simulink model "CruiseControl_pp_harness_ReqProve"  (R2016a)
settings: Solver=ode3  StartTime=0  StopTime=0.40000000000000002  FixedStep=0.10000000000000001  RelTol=1e-3
PreLoadFcn:
  | CruiseControl_dd;
  | definePPenums;
undefined symbols (not defined in the file or in its folder): mintspeed, sigbuilder_block
libraries: sldvlib x20, simulink x8
settings Model: SldvGeneratedHarnessModel=TestUnitModel=CruiseControl_pp|  Creator=The MathWorks Inc.  LastModifiedBy=colosky
settings DataIOCC: LimitDataPoints=on  SaveFormat=StructureWithTime  SaveOutput=off  SaveTime=off
settings OptimizationCC: BlockReduction=off  DefaultParameterBehavior=Inlined  InlineInvariantSignals=on  ExpressionFolding=off  ExpressionDepthLimit=2147483647  InitFltsAndDblsToZero=on  OptimizeModelRefInitCode=on  LifeSpan=1
settings DebuggingCC: SaveWithParameterizedLinksMsg=none  UnderspecifiedInitializationDetection=Classic  MergeDetectMultiDrivingBlocksExec=none  SolverPrmCheckMsg=warning  InheritedTsInSrcMsg=none  FcnCallInpInsideContextMsg=UseLocalSettings  AllowSymbolicDim=off  StateNameClashWarn=warning  StrictBusMsg=ErrorOnBusTreatedAsVector
settings HardwareCC: ProdBitPerPointer=32  ProdLargestAtomicFloat=None  ProdEndianess=Unspecified  ProdWordSize=32  ProdHWDeviceType=32-bit Generic
settings ModelReferenceCC: ModelReferenceNumInstancesAllowed=Single  PropagateSignalLabelsOutOfModel=off
settings SFSimCC: SimParseCustomCode=off
settings RTWCC: SystemTargetFile=ert.tlc  TemplateMakefile=ert_default_tmf  GenerateReport=on  IncludeHyperlinkInReport=on  LaunchReport=on  GenerateTraceInfo=on  GenerateTraceReport=on  GenerateTraceReportSl=on  GenerateTraceReportSf=on  GenerateTraceReportEml=on
settings CodeAppCC: ForceParamTrailComments=on  IgnoreCustomStorageClasses=off  OperatorAnnotations=on  SimulinkDataObjDesc=on  SFDataObjDesc=on  MATLABFcnDesc=on  InsertBlockDesc=on  MATLABSourceComments=on
settings ERTTargetCC: GenerateSampleERTMain=on  InlinedParameterPlacement=NonHierarchical  ERTCustomFileTemplate=example_file_process.tlc
settings ConfigComp: CovMetricSettings=dcme  CovHtmlReporting=off  CovSaveCumulativeToWorkspaceVar=off  CovSaveSingleToWorkspaceVar=off  CovModelRefEnable=Off  CovSFcnEnable=off  DVMode=PropertyProving  DVMaxProcessTime=3000  DVDisplayUnsatisfiableObjectives=on  DVAutomaticStubbing=off  DVMakeOutputFilesUnique=off  DVParameters=on  DVParametersUseConfig=on  DVModelCoverageObjectives=MCDC  DVMaxTestCaseSteps=500  DVTestSuiteOptimization=CombinedObjectives  DVAssertions=EnableAll  DVProofAssumptions=EnableAll  DVDetectIntegerOverflow=off  DVDetectActiveLogic=on  DVMaxViolationSteps=10  DVSaveDataFile=off  DVReportIncludeGraphics=on  DVDisplayResultsOnModel=on

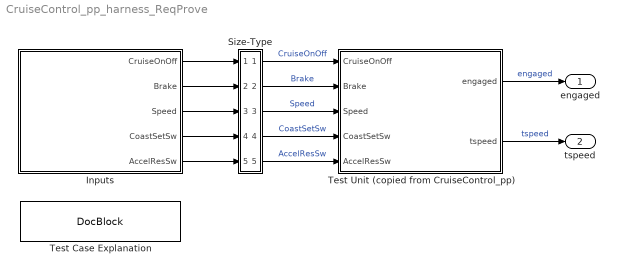
== system CruiseControl_pp_harness_ReqProve ==
  Inputs : Subsystem  Tag=STV Subsys  LoadFcn=sigbuilder_block('load',[50 50 520 400 ]);  StartFcn=sigbuilder_block('start');  StopFcn=sigbuilder_block('stop');  ClipboardFcn=sigbuilder_block('clipboard');  mask(Sigbuilder block){}
      mask init:
      | if ~strcmp(get_param(bdroot(gcb),'SimulationStatus'),'stopped'),tuvar = sigbuilder_block('maskInit'); end
      settings: CopyFcn=sigbuilder_block('copy');  DeleteFcn=sigbuilder_block('delete');  ModelCloseFcn=sigbuilder_block('modelClose');  PreSaveFcn=sigbuilder_block('preSave');  PauseFcn=sigbuilder_block('pause');  ContinueFcn=sigbuilder_block('continue');  NameChangeFcn=sigbuilder_block('namechange');  OpenFcn=sigbuilder_block('open');  CloseFcn=sigbuilder_block('close');
      mask Display: plot(0, 0, 100, 100,[2, 2, 32, 32, 2], [68, 8, 8, 68, 68],[32, 2], [38, 38], [32, 19, 2],[53, 60, 44], [32, 17, 17, 2],[16, 16, 31, 31]);txt = getActiveGroup(gcbh);text(2, 100, txt,'verticalAlignment', 'top');
  Size-Type : Subsystem
  Test Case Explanation : simulink/Model-Wide Utilities/DocBlock  DocumentType=Text
  Test Unit (copied from CruiseControl_pp) : Subsystem
  engaged : Outport  OutDataTypeStr=boolean  PortDimensions=1
  tspeed : Outport  Port=2  OutDataTypeStr=uint8  PortDimensions=1
  wires:
  Inputs/1(CruiseOnOff) -> Size-Type/1(In1)
  Size-Type/1(Out1) -> Test Unit (copied from CruiseControl_pp)/1(CruiseOnOff)  "CruiseOnOff"
  Inputs/2(Brake) -> Size-Type/2(In2)
  Size-Type/2(Out2) -> Test Unit (copied from CruiseControl_pp)/2(Brake)  "Brake"
  Inputs/3(Speed) -> Size-Type/3(In3)
  Size-Type/3(Out3) -> Test Unit (copied from CruiseControl_pp)/3(Speed)  "Speed"
  Inputs/4(CoastSetSw) -> Size-Type/4(In4)
  Size-Type/4(Out4) -> Test Unit (copied from CruiseControl_pp)/4(CoastSetSw)  "CoastSetSw"
  Inputs/5(AccelResSw) -> Size-Type/5(In5)
  Size-Type/5(Out5) -> Test Unit (copied from CruiseControl_pp)/5(AccelResSw)  "AccelResSw"
  Test Unit (copied from CruiseControl_pp)/1(engaged) -> engaged/1  "engaged"
  Test Unit (copied from CruiseControl_pp)/2(tspeed) -> tspeed/1  "tspeed"

== system CruiseControl_pp_harness_ReqProve/Inputs ==
  Demux : Demux  Tag=STV Demux  Outputs=5
  FromWs : FromWorkspace  Tag=STV FromWs  VariableName=tuvar  SampleTime=0
      SigBuilderData=|
      | dataSet.timeRange = [0 0.4]
      | dataSet.name = 'Counterexample 1'
      | sbobj.Name = 'Signal Builder'
      | sbobj.Groups.Name = 'Counterexample 1'
      | sbobj.Groups.Signals(1).Name = 'CruiseOnOff'
      | sbobj.Groups.Signals(1).XData = [0 0.1 0.2 0.3 0.4]
      | sbobj.Groups.Signals(1).YData = [1 1 1 1 1]
      | sbobj.Groups.Signals(2).Name = 'Brake'
      | sbobj.Groups.Signals(2).XData = [0 0.1 0.1 0.2 0.2 0.3 0.3 0.4]
      | sbobj.Groups.Signals(2).YData = [0 0 0 0 0 0 0 0]
      | sbobj.Groups.Signals(3).Name = 'Speed'
      | sbobj.Groups.Signals(3).XData = [0 0.1 0.1 0.2 0.2 0.3 0.3 0.4]
      | sbobj.Groups.Signals(3).YData = [48 48 52 52 27 27 52 52]
      | sbobj.Groups.Signals(4).Name = 'CoastSetSw'
      | sbobj.Groups.Signals(4).XData = [0 0.1 0.1 0.2 0.2 0.3 0.3 0.4]
      | sbobj.Groups.Signals(4).YData = [0 0 0 0 1 1 1 1]
      | sbobj.Groups.Signals(5).Name = 'AccelResSw'
      | sbobj.Groups.Signals(5).XData = [0 0.1 0.1 0.2 0.2 0.3 0.3 0.4]
      | sbobj.Groups.Signals(5).YData = [1 1 1 1 0 0 1 1]
      | sbobj.Groups.TimeRange = [0 0.4]
  CruiseOnOff : Outport  Tag=STV Outport
  Brake : Outport  Tag=STV Outport  Port=2
  Speed : Outport  Tag=STV Outport  Port=3
  CoastSetSw : Outport  Tag=STV Outport  Port=4
  AccelResSw : Outport  Tag=STV Outport  Port=5
  wires:
  FromWs/1 -> Demux/1
  Demux/1 -> CruiseOnOff/1
  Demux/2 -> Brake/1
  Demux/3 -> Speed/1
  Demux/4 -> CoastSetSw/1
  Demux/5 -> AccelResSw/1

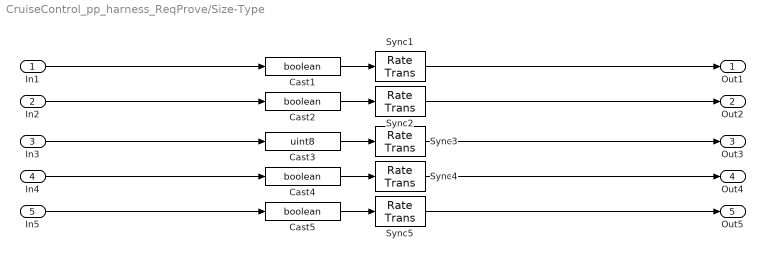
== system CruiseControl_pp_harness_ReqProve/Size-Type ==
  In1 : Inport
  In2 : Inport  Port=2
  In3 : Inport  Port=3
  In4 : Inport  Port=4
  In5 : Inport  Port=5
  Cast{1..2,4..5} (4 alike) : DataTypeConversion  OutDataTypeStr=boolean  RndMeth=Nearest  SaturateOnIntegerOverflow=on
  Cast3 : DataTypeConversion  OutDataTypeStr=uint8  RndMeth=Nearest  SaturateOnIntegerOverflow=on
  Sync{1..5} (5 alike) : RateTransition  OutPortSampleTime=[0.10000000000000001,0]
  Out1 : Outport
  Out2 : Outport  Port=2
  Out3 : Outport  Port=3
  Out4 : Outport  Port=4
  Out5 : Outport  Port=5
  wires:
  In1/1 -> Cast1/1
  Cast1/1 -> Sync1/1
  Sync1/1 -> Out1/1
  In2/1 -> Cast2/1
  Cast2/1 -> Sync2/1
  Sync2/1 -> Out2/1
  In3/1 -> Cast3/1
  Cast3/1 -> Sync3/1
  Sync3/1 -> Out3/1
  In4/1 -> Cast4/1
  Cast4/1 -> Sync4/1
  Sync4/1 -> Out4/1
  In5/1 -> Cast5/1
  Cast5/1 -> Sync5/1
  Sync5/1 -> Out5/1

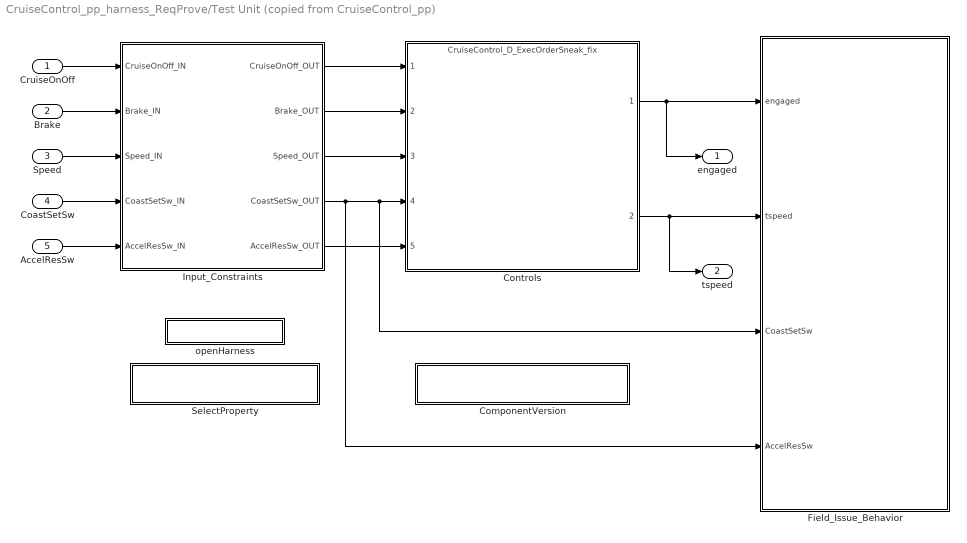
== system CruiseControl_pp_harness_ReqProve/Test Unit (copied from CruiseControl_pp) ==
  CruiseOnOff : Inport  OutDataTypeStr=boolean  PortDimensions=1
  Brake : Inport  Port=2  OutDataTypeStr=boolean  PortDimensions=1
  Speed : Inport  Port=3  OutDataTypeStr=uint8  PortDimensions=1
  CoastSetSw : Inport  Port=4  OutDataTypeStr=boolean  PortDimensions=1
  AccelResSw : Inport  Port=5  OutDataTypeStr=boolean  PortDimensions=1
  ComponentVersion : Subsystem  mask(ControlsVersion){}
      mask help: Selects the block choice for the "Controls" subystem.
      settings: OpenFcn=|
      | [~,enumVers] = enumeration('CtrlsVerEnum');
      | [selection, ok] = listdlg('Name','Component Version','ListSize',[210 110],'SelectionMode','single', ...
      |    'PromptString','Select Cruise Control version...','ListString',enumVers,'InitialValue',uint32(CtrlsVer));
      | waitfor(selection);
      | if ok
      |    CtrlsVer = CtrlsVerEnum(enumVers{selection});
      | end
      mask Display: disp('Select Cruise Control version to verify...');
  Controls : ModelReference  ModelNameDialog=CruiseControl_D_ExecOrderSneak_fix.slx  SimulationMode=Normal  Variant=on  ModelReferenceVersion=1.515
  Field_Issue_Behavior : Subsystem  Variant=on
      settings: AttributesFormatString=%<BlockChoice>
  Input_Constraints : Subsystem  Variant=on
      settings: AttributesFormatString=%<BlockChoice>
  SelectProperty : Subsystem  mask(PropertySelection){}
      mask help: Selects the block choice for the "Input_Constraints" and "Field_Issue_Behavior" subystems.
      settings: OpenFcn=|
      | [~,enumProps] = enumeration('PropEnum');
      | [selection, ok] = listdlg('Name','Propery To Prove','ListSize',[210 110],'SelectionMode','single', ...
      |    'PromptString','Select Property to Prove...','ListString',enumProps,'InitialValue',uint32(Prop2Prove));
      | waitfor(selection);
      | if ok
      |    Prop2Prove = PropEnum(enumProps{selection});
      | end
      mask DialogControl DescGroupVar Prompt: Description
      mask Display: disp('Selected Property to Prove...');
  openHarness : Subsystem
      settings: OpenFcn=|
      | switch (CtrlsVer)
      | case CtrlsVerEnum.CtrlC_ExecOrder_fix
      |     load_PP_harness('CruiseControl_pp_harness_FieldIssue');
      | case CtrlsVerEnum.CtrlD_ExecOrderSneak_fix
      |     load_PP_harness('CruiseControl_pp_harness_ReqProve');
      | case CtrlsVerEnum.CtrlE_ExecOrderSneakDblReject_fix
      |     load_PP_harness('CruiseControl_pp_harness_ReqWithParsProve');
      | end
      mask Display: disp(['Open Harness']);
  engaged : Outport  OutDataTypeStr=boolean  PortDimensions=1
  tspeed : Outport  Port=2  OutDataTypeStr=uint8  PortDimensions=1
  wires:
  Controls/2 -> Field_Issue_Behavior/2(tspeed), tspeed/1
  AccelResSw/1 -> Input_Constraints/5(AccelResSw_IN)
  Speed/1 -> Input_Constraints/3(Speed_IN)
  CruiseOnOff/1 -> Input_Constraints/1(CruiseOnOff_IN)
  Brake/1 -> Input_Constraints/2(Brake_IN)
  CoastSetSw/1 -> Input_Constraints/4(CoastSetSw_IN)
  Input_Constraints/1(CruiseOnOff_OUT) -> Controls/1
  Input_Constraints/2(Brake_OUT) -> Controls/2
  Input_Constraints/3(Speed_OUT) -> Controls/3
  Input_Constraints/4(CoastSetSw_OUT) -> Controls/4, Field_Issue_Behavior/3(CoastSetSw), Field_Issue_Behavior/4(AccelResSw)
  Input_Constraints/5(AccelResSw_OUT) -> Controls/5
  Controls/1 -> Field_Issue_Behavior/1(engaged), engaged/1

== system CruiseControl_pp_harness_ReqProve/Test Unit (copied from CruiseControl_pp)/ComponentVersion ==

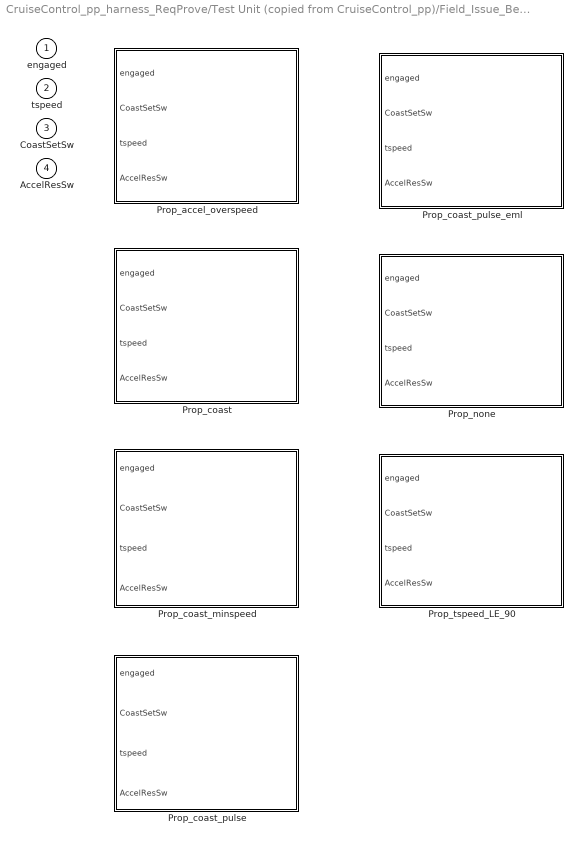
== system CruiseControl_pp_harness_ReqProve/Test Unit (copied from CruiseControl_pp)/Field_Issue_Behavior ==
  engaged : Inport
  tspeed : Inport  Port=2
  CoastSetSw : Inport  Port=3
  AccelResSw : Inport  Port=4
  Prop_accel_overspeed : Subsystem  VariantControl=Prop2Prove == PropEnum.Prop_accel_overspeed
  Prop_coast : Subsystem  VariantControl=Prop2Prove == PropEnum.Prop_coast
  Prop_coast_minspeed : Subsystem  VariantControl=Prop2Prove == PropEnum.Prop_coast_minspeed
  Prop_coast_pulse : Subsystem  VariantControl=Prop2Prove == PropEnum.Prop_coast_pulse
  Prop_coast_pulse_eml : Subsystem  VariantControl=Prop2Prove == PropEnum.Prop_coast_pulse_eml
  Prop_none : Subsystem  VariantControl=Prop2Prove == PropEnum.Prop_none
  Prop_tspeed_LE_90 : Subsystem  VariantControl=Prop2Prove == PropEnum.Prop_tspeed_LE_90

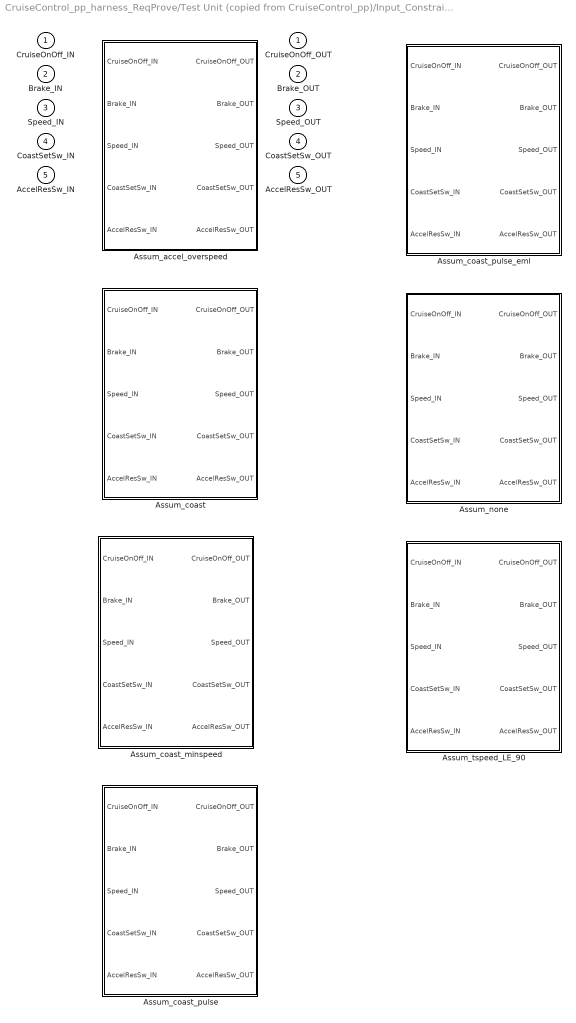
== system CruiseControl_pp_harness_ReqProve/Test Unit (copied from CruiseControl_pp)/Input_Constraints ==
  CruiseOnOff_IN : Inport
  Brake_IN : Inport  Port=2
  Speed_IN : Inport  Port=3
  CoastSetSw_IN : Inport  Port=4
  AccelResSw_IN : Inport  Port=5
  Assum_accel_overspeed : Subsystem  VariantControl=Prop2Prove == PropEnum.Prop_accel_overspeed
  Assum_coast : Subsystem  VariantControl=Prop2Prove == PropEnum.Prop_coast
  Assum_coast_minspeed : Subsystem  VariantControl=Prop2Prove == PropEnum.Prop_coast_minspeed
  Assum_coast_pulse : Subsystem  VariantControl=Prop2Prove == PropEnum.Prop_coast_pulse
  Assum_coast_pulse_eml : Subsystem  VariantControl=Prop2Prove == PropEnum.Prop_coast_pulse_eml
  Assum_none : Subsystem  VariantControl=Prop2Prove == PropEnum.Prop_none
  Assum_tspeed_LE_90 : Subsystem  VariantControl=Prop2Prove == PropEnum.Prop_tspeed_LE_90
  CruiseOnOff_OUT : Outport
  Brake_OUT : Outport  Port=2
  Speed_OUT : Outport  Port=3
  CoastSetSw_OUT : Outport  Port=4
  AccelResSw_OUT : Outport  Port=5

== system CruiseControl_pp_harness_ReqProve/Test Unit (copied from CruiseControl_pp)/SelectProperty ==

== system CruiseControl_pp_harness_ReqProve/Test Unit (copied from CruiseControl_pp)/openHarness ==

== system CruiseControl_pp_harness_ReqProve/Test Unit (copied from CruiseControl_pp)/Field_Issue_Behavior/Prop_accel_overspeed ==
  engaged : Inport
  CoastSetSw : Inport  Port=2
  tspeed : Inport  Port=3
  AccelResSw : Inport  Port=4
  Compare To Constant : simulink/Logic and Bit Operations/Compare To Constant  relop=<=  const=95  OutDataTypeStr=boolean
  EngagedImplies : sldvlib/Verification Utilities/Implies
  Logical Operator2 : Logic  AllPortsSameDT=off  OutDataTypeStr=boolean
  Prop_accel_overspeed : sldvlib/Objectives and Constraints/Proof Objective  enabled=on  customAVTBlockType=Proof Objective  intervals=true  dispValues=on  outEnabled=off  enableStopSim=off
      settings: AttributesFormatString=%<intervals>
  Terminator1 : Terminator
  wires:
  EngagedImplies/1 -> Prop_accel_overspeed/1
  Logical Operator2/1 -> EngagedImplies/1
  AccelResSw/1 -> Logical Operator2/2
  engaged/1 -> Logical Operator2/1
  Compare To Constant/1 -> EngagedImplies/2
  tspeed/1 -> Compare To Constant/1
  CoastSetSw/1 -> Terminator1/1

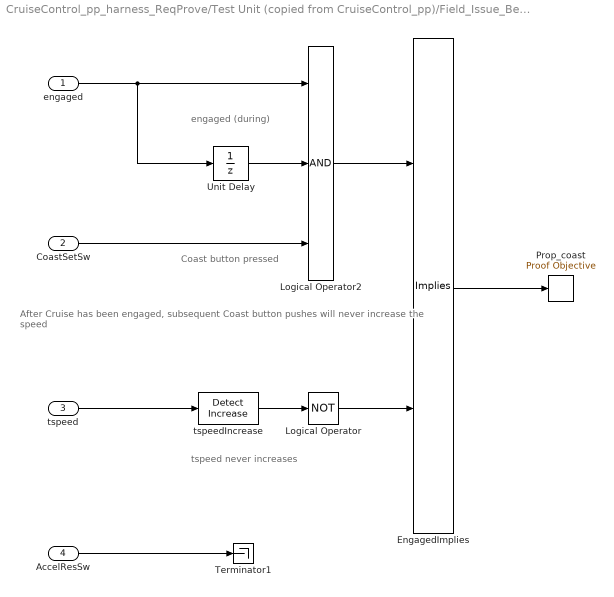
== system CruiseControl_pp_harness_ReqProve/Test Unit (copied from CruiseControl_pp)/Field_Issue_Behavior/Prop_coast ==
  note: After Cruise has been engaged, subsequent Coast button pushes will never increase the speed
  note: Coast button pressed
  note: tspeed never increases
  note: engaged (during)
  engaged : Inport
  CoastSetSw : Inport  Port=2
  tspeed : Inport  Port=3
  AccelResSw : Inport  Port=4
  EngagedImplies : sldvlib/Verification Utilities/Implies
  Logical Operator : Logic  Operator=NOT  AllPortsSameDT=off  OutDataTypeStr=boolean
  Logical Operator2 : Logic  Inputs=3  AllPortsSameDT=off  OutDataTypeStr=boolean
  Prop_coast : sldvlib/Objectives and Constraints/Proof Objective  enabled=on  customAVTBlockType=Proof Objective  intervals=true  dispValues=on  outEnabled=off  enableStopSim=off
      settings: AttributesFormatString=%<intervals>
  Terminator1 : Terminator
  Unit Delay : UnitDelay  SampleTime=-1
  tspeedIncrease : simulink/Logic and Bit Operations/Detect Increase  vinit=0.0  InputProcessing=Inherited  OutDataTypeStr=boolean
  wires:
  EngagedImplies/1 -> Prop_coast/1
  tspeedIncrease/1 -> Logical Operator/1
  tspeed/1 -> tspeedIncrease/1
  Unit Delay/1 -> Logical Operator2/2
  AccelResSw/1 -> Terminator1/1
  engaged/1 -> Logical Operator2/1, Unit Delay/1
  Logical Operator/1 -> EngagedImplies/2
  CoastSetSw/1 -> Logical Operator2/3
  Logical Operator2/1 -> EngagedImplies/1

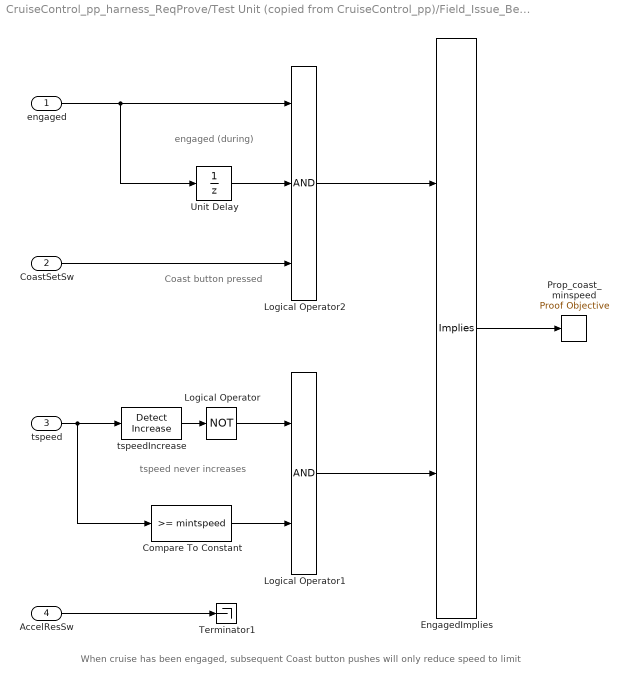
== system CruiseControl_pp_harness_ReqProve/Test Unit (copied from CruiseControl_pp)/Field_Issue_Behavior/Prop_coast_minspeed ==
  note: When cruise has been engaged, subsequent Coast button pushes will only reduce speed to limit
  note: Coast button pressed
  note: tspeed never increases
  note: engaged (during)
  engaged : Inport
  CoastSetSw : Inport  Port=2
  tspeed : Inport  Port=3
  AccelResSw : Inport  Port=4
  Compare To Constant : simulink/Logic and Bit Operations/Compare To Constant  relop=>=  const=mintspeed  OutDataTypeStr=boolean
  EngagedImplies : sldvlib/Verification Utilities/Implies
  Logical Operator : Logic  Operator=NOT  AllPortsSameDT=off  OutDataTypeStr=boolean
  Logical Operator1 : Logic  AllPortsSameDT=off  OutDataTypeStr=boolean
  Logical Operator2 : Logic  Inputs=3  AllPortsSameDT=off  OutDataTypeStr=boolean
  Prop_coast_minspeed : sldvlib/Objectives and Constraints/Proof Objective  enabled=on  customAVTBlockType=Proof Objective  intervals=true  dispValues=on  outEnabled=off  enableStopSim=off
      settings: AttributesFormatString=%<intervals>
  Terminator1 : Terminator
  Unit Delay : UnitDelay  SampleTime=-1
  tspeedIncrease : simulink/Logic and Bit Operations/Detect Increase  vinit=0.0  InputProcessing=Inherited  OutDataTypeStr=boolean
  wires:
  Logical Operator1/1 -> EngagedImplies/2
  Compare To Constant/1 -> Logical Operator1/2
  Logical Operator/1 -> Logical Operator1/1
  EngagedImplies/1 -> Prop_coast_minspeed/1
  tspeedIncrease/1 -> Logical Operator/1
  tspeed/1 -> tspeedIncrease/1, Compare To Constant/1
  Unit Delay/1 -> Logical Operator2/2
  AccelResSw/1 -> Terminator1/1
  engaged/1 -> Logical Operator2/1, Unit Delay/1
  CoastSetSw/1 -> Logical Operator2/3
  Logical Operator2/1 -> EngagedImplies/1

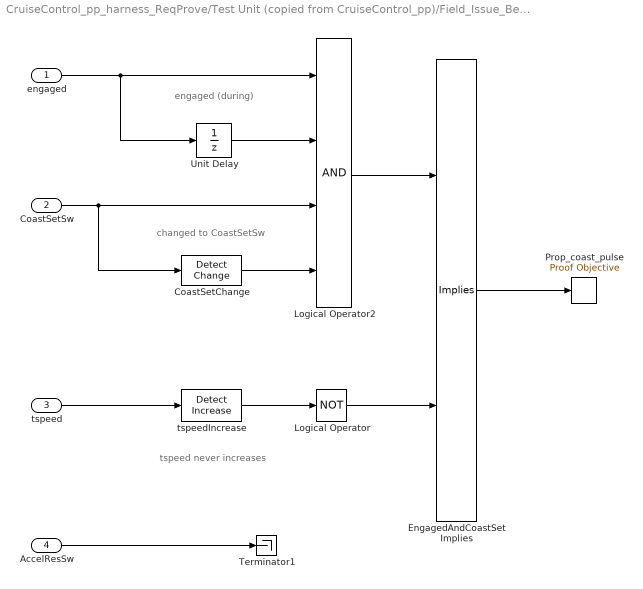
== system CruiseControl_pp_harness_ReqProve/Test Unit (copied from CruiseControl_pp)/Field_Issue_Behavior/Prop_coast_pulse ==
  note: engaged (during)
  note: tspeed never increases
  note: changed to CoastSetSw
  engaged : Inport
  CoastSetSw : Inport  Port=2
  tspeed : Inport  Port=3
  AccelResSw : Inport  Port=4
  CoastSetChange : simulink/Logic and Bit Operations/Detect Change  vinit=0  InputProcessing=Inherited  OutDataTypeStr=boolean
  EngagedAndCoastSetImplies : sldvlib/Verification Utilities/Implies
  Logical Operator : Logic  Operator=NOT  AllPortsSameDT=off  OutDataTypeStr=boolean
  Logical Operator2 : Logic  Inputs=4  AllPortsSameDT=off  OutDataTypeStr=boolean
  Prop_coast_pulse : sldvlib/Objectives and Constraints/Proof Objective  enabled=on  customAVTBlockType=Proof Objective  intervals=true  dispValues=on  outEnabled=off  enableStopSim=off
      settings: AttributesFormatString=%<intervals>
  Terminator1 : Terminator
  Unit Delay : UnitDelay  SampleTime=-1
  tspeedIncrease : simulink/Logic and Bit Operations/Detect Increase  vinit=0.0  InputProcessing=Inherited  OutDataTypeStr=boolean
  wires:
  CoastSetChange/1 -> Logical Operator2/4
  Unit Delay/1 -> Logical Operator2/2
  engaged/1 -> Logical Operator2/1, Unit Delay/1
  EngagedAndCoastSetImplies/1 -> Prop_coast_pulse/1
  tspeedIncrease/1 -> Logical Operator/1
  AccelResSw/1 -> Terminator1/1
  Logical Operator2/1 -> EngagedAndCoastSetImplies/1
  tspeed/1 -> tspeedIncrease/1
  CoastSetSw/1 -> CoastSetChange/1, Logical Operator2/3
  Logical Operator/1 -> EngagedAndCoastSetImplies/2

== system CruiseControl_pp_harness_ReqProve/Test Unit (copied from CruiseControl_pp)/Field_Issue_Behavior/Prop_coast_pulse_eml ==
  engaged : Inport
  CoastSetSw : Inport  Port=2
  tspeed : Inport  Port=3
  AccelResSw : Inport  Port=4
  MATLAB Function : Subsystem  TreatAsAtomicUnit=on
  Porp_coast_pulse_eml : sldvlib/Objectives and Constraints/Proof Objective  enabled=on  customAVTBlockType=Proof Objective  intervals=true  dispValues=on  outEnabled=off  enableStopSim=off
      settings: AttributesFormatString=%<intervals>
  Terminator1 : Terminator
  wires:
  MATLAB Function/1(property) -> Porp_coast_pulse_eml/1
  tspeed/1 -> MATLAB Function/3(tspeed)
  CoastSetSw/1 -> MATLAB Function/2(CoastSetSw)
  engaged/1 -> MATLAB Function/1(engaged)
  AccelResSw/1 -> Terminator1/1

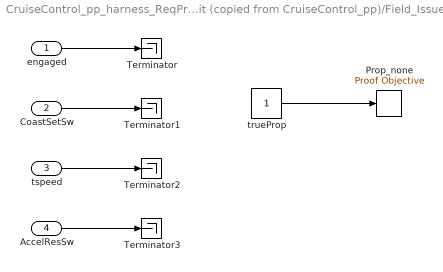
== system CruiseControl_pp_harness_ReqProve/Test Unit (copied from CruiseControl_pp)/Field_Issue_Behavior/Prop_none ==
  engaged : Inport
  CoastSetSw : Inport  Port=2
  tspeed : Inport  Port=3
  AccelResSw : Inport  Port=4
  Prop_none : sldvlib/Objectives and Constraints/Proof Objective  enabled=on  customAVTBlockType=Proof Objective  intervals=true  dispValues=on  outEnabled=off  enableStopSim=off
      settings: AttributesFormatString=%<intervals>
  Terminator{,1..3} (4 alike) : Terminator
  trueProp : Constant  OutDataTypeStr=boolean
  wires:
  trueProp/1 -> Prop_none/1
  AccelResSw/1 -> Terminator3/1
  engaged/1 -> Terminator/1
  tspeed/1 -> Terminator2/1
  CoastSetSw/1 -> Terminator1/1

== system CruiseControl_pp_harness_ReqProve/Test Unit (copied from CruiseControl_pp)/Field_Issue_Behavior/Prop_tspeed_LE_90 ==
  engaged : Inport
  CoastSetSw : Inport  Port=2
  tspeed : Inport  Port=3
  AccelResSw : Inport  Port=4
  Compare To Constant : simulink/Logic and Bit Operations/Compare To Constant  relop=<=  const=90  OutDataTypeStr=boolean
  Prop_tspeed_LE_90 : sldvlib/Objectives and Constraints/Proof Objective  enabled=on  customAVTBlockType=Proof Objective  intervals=true  dispValues=on  outEnabled=off  enableStopSim=off
      settings: AttributesFormatString=%<intervals>
  Terminator : Terminator
  Terminator1 : Terminator
  Terminator2 : Terminator
  wires:
  Compare To Constant/1 -> Prop_tspeed_LE_90/1
  AccelResSw/1 -> Terminator2/1
  CoastSetSw/1 -> Terminator1/1
  tspeed/1 -> Compare To Constant/1
  engaged/1 -> Terminator/1

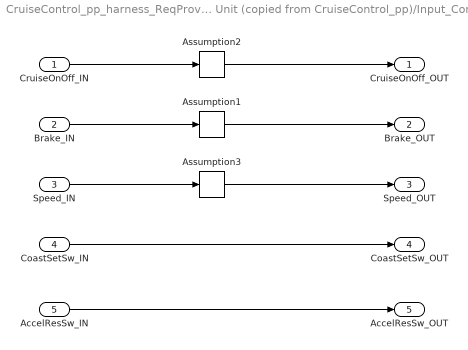
== system CruiseControl_pp_harness_ReqProve/Test Unit (copied from CruiseControl_pp)/Input_Constraints/Assum_accel_overspeed ==
  CruiseOnOff_IN : Inport  OutDataTypeStr=boolean  PortDimensions=1
  Brake_IN : Inport  Port=2  OutDataTypeStr=boolean  PortDimensions=1
  Speed_IN : Inport  Port=3  OutDataTypeStr=uint8  PortDimensions=1
  CoastSetSw_IN : Inport  Port=4  OutDataTypeStr=boolean  PortDimensions=1
  AccelResSw_IN : Inport  Port=5  OutDataTypeStr=boolean  PortDimensions=1
  Assumption1 : sldvlib/Objectives and Constraints/Assumption  enabled=on  customAVTBlockType=Assumption  intervals=false  initial=off  dispValues=on  outEnabled=on
      settings: AttributesFormatString=%<intervals>
  Assumption2 : sldvlib/Objectives and Constraints/Assumption  enabled=on  customAVTBlockType=Assumption  intervals=true  initial=off  dispValues=on  outEnabled=on
      settings: AttributesFormatString=%<intervals>
  Assumption3 : sldvlib/Objectives and Constraints/Assumption  enabled=on  customAVTBlockType=Assumption  intervals={[88 Inf]}  initial=off  dispValues=on  outEnabled=on
      settings: AttributesFormatString=%<intervals>
  CruiseOnOff_OUT : Outport
  Brake_OUT : Outport  Port=2
  Speed_OUT : Outport  Port=3
  CoastSetSw_OUT : Outport  Port=4
  AccelResSw_OUT : Outport  Port=5
  wires:
  Assumption3/1 -> Speed_OUT/1
  Assumption1/1 -> Brake_OUT/1
  Assumption2/1 -> CruiseOnOff_OUT/1
  CruiseOnOff_IN/1 -> Assumption2/1
  Brake_IN/1 -> Assumption1/1
  AccelResSw_IN/1 -> AccelResSw_OUT/1
  CoastSetSw_IN/1 -> CoastSetSw_OUT/1
  Speed_IN/1 -> Assumption3/1

== system CruiseControl_pp_harness_ReqProve/Test Unit (copied from CruiseControl_pp)/Input_Constraints/Assum_coast ==
  CruiseOnOff_IN : Inport  OutDataTypeStr=boolean  PortDimensions=1
  Brake_IN : Inport  Port=2  OutDataTypeStr=boolean  PortDimensions=1
  Speed_IN : Inport  Port=3  OutDataTypeStr=uint8  PortDimensions=1
  CoastSetSw_IN : Inport  Port=4  OutDataTypeStr=boolean  PortDimensions=1
  AccelResSw_IN : Inport  Port=5  OutDataTypeStr=boolean  PortDimensions=1
  CruiseOnOff_OUT : Outport
  Brake_OUT : Outport  Port=2
  Speed_OUT : Outport  Port=3
  CoastSetSw_OUT : Outport  Port=4
  AccelResSw_OUT : Outport  Port=5
  wires:
  AccelResSw_IN/1 -> AccelResSw_OUT/1
  Brake_IN/1 -> Brake_OUT/1
  CruiseOnOff_IN/1 -> CruiseOnOff_OUT/1
  Speed_IN/1 -> Speed_OUT/1
  CoastSetSw_IN/1 -> CoastSetSw_OUT/1

== system CruiseControl_pp_harness_ReqProve/Test Unit (copied from CruiseControl_pp)/Input_Constraints/Assum_coast_minspeed ==
  CruiseOnOff_IN : Inport  OutDataTypeStr=boolean  PortDimensions=1
  Brake_IN : Inport  Port=2  OutDataTypeStr=boolean  PortDimensions=1
  Speed_IN : Inport  Port=3  OutDataTypeStr=uint8  PortDimensions=1
  CoastSetSw_IN : Inport  Port=4  OutDataTypeStr=boolean  PortDimensions=1
  AccelResSw_IN : Inport  Port=5  OutDataTypeStr=boolean  PortDimensions=1
  CruiseOnOff_OUT : Outport
  Brake_OUT : Outport  Port=2
  Speed_OUT : Outport  Port=3
  CoastSetSw_OUT : Outport  Port=4
  AccelResSw_OUT : Outport  Port=5
  wires:
  AccelResSw_IN/1 -> AccelResSw_OUT/1
  Brake_IN/1 -> Brake_OUT/1
  CruiseOnOff_IN/1 -> CruiseOnOff_OUT/1
  Speed_IN/1 -> Speed_OUT/1
  CoastSetSw_IN/1 -> CoastSetSw_OUT/1

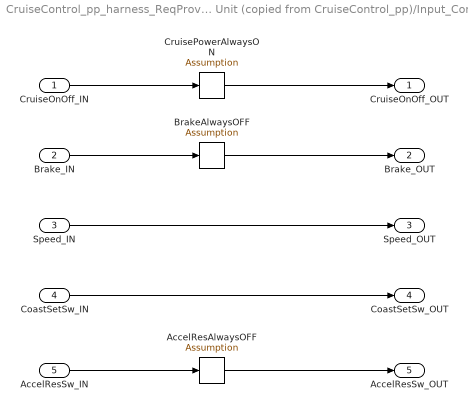
== system CruiseControl_pp_harness_ReqProve/Test Unit (copied from CruiseControl_pp)/Input_Constraints/Assum_coast_pulse ==
  CruiseOnOff_IN : Inport  OutDataTypeStr=boolean  PortDimensions=1
  Brake_IN : Inport  Port=2  OutDataTypeStr=boolean  PortDimensions=1
  Speed_IN : Inport  Port=3  OutDataTypeStr=uint8  PortDimensions=1
  CoastSetSw_IN : Inport  Port=4  OutDataTypeStr=boolean  PortDimensions=1
  AccelResSw_IN : Inport  Port=5  OutDataTypeStr=boolean  PortDimensions=1
  AccelResAlwaysOFF : sldvlib/Objectives and Constraints/Assumption  enabled=on  customAVTBlockType=Assumption  intervals=false  initial=off  dispValues=on  outEnabled=on
      settings: AttributesFormatString=%<intervals>
  BrakeAlwaysOFF : sldvlib/Objectives and Constraints/Assumption  enabled=on  customAVTBlockType=Assumption  intervals=false  initial=off  dispValues=on  outEnabled=on
      settings: AttributesFormatString=%<intervals>
  CruisePowerAlwaysON : sldvlib/Objectives and Constraints/Assumption  enabled=on  customAVTBlockType=Assumption  intervals=true  initial=off  dispValues=on  outEnabled=on
      settings: AttributesFormatString=%<intervals>
  CruiseOnOff_OUT : Outport
  Brake_OUT : Outport  Port=2
  Speed_OUT : Outport  Port=3
  CoastSetSw_OUT : Outport  Port=4
  AccelResSw_OUT : Outport  Port=5
  wires:
  CoastSetSw_IN/1 -> CoastSetSw_OUT/1
  AccelResSw_IN/1 -> AccelResAlwaysOFF/1
  Speed_IN/1 -> Speed_OUT/1
  Brake_IN/1 -> BrakeAlwaysOFF/1
  CruiseOnOff_IN/1 -> CruisePowerAlwaysON/1
  CruisePowerAlwaysON/1 -> CruiseOnOff_OUT/1
  BrakeAlwaysOFF/1 -> Brake_OUT/1
  AccelResAlwaysOFF/1 -> AccelResSw_OUT/1

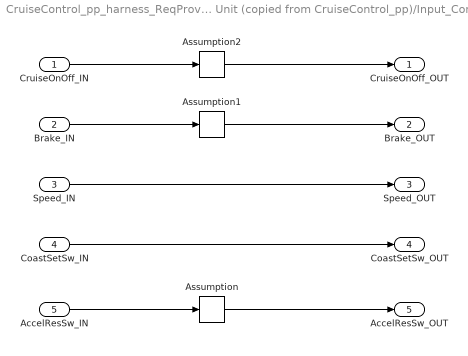
== system CruiseControl_pp_harness_ReqProve/Test Unit (copied from CruiseControl_pp)/Input_Constraints/Assum_coast_pulse_eml ==
  CruiseOnOff_IN : Inport  OutDataTypeStr=boolean  PortDimensions=1
  Brake_IN : Inport  Port=2  OutDataTypeStr=boolean  PortDimensions=1
  Speed_IN : Inport  Port=3  OutDataTypeStr=uint8  PortDimensions=1
  CoastSetSw_IN : Inport  Port=4  OutDataTypeStr=boolean  PortDimensions=1
  AccelResSw_IN : Inport  Port=5  OutDataTypeStr=boolean  PortDimensions=1
  Assumption : sldvlib/Objectives and Constraints/Assumption  enabled=on  customAVTBlockType=Assumption  intervals=false  initial=off  dispValues=on  outEnabled=on
      settings: AttributesFormatString=%<intervals>
  Assumption1 : sldvlib/Objectives and Constraints/Assumption  enabled=on  customAVTBlockType=Assumption  intervals=false  initial=off  dispValues=on  outEnabled=on
      settings: AttributesFormatString=%<intervals>
  Assumption2 : sldvlib/Objectives and Constraints/Assumption  enabled=on  customAVTBlockType=Assumption  intervals=true  initial=off  dispValues=on  outEnabled=on
      settings: AttributesFormatString=%<intervals>
  CruiseOnOff_OUT : Outport
  Brake_OUT : Outport  Port=2
  Speed_OUT : Outport  Port=3
  CoastSetSw_OUT : Outport  Port=4
  AccelResSw_OUT : Outport  Port=5
  wires:
  Assumption/1 -> AccelResSw_OUT/1
  Assumption1/1 -> Brake_OUT/1
  Assumption2/1 -> CruiseOnOff_OUT/1
  CruiseOnOff_IN/1 -> Assumption2/1
  Brake_IN/1 -> Assumption1/1
  Speed_IN/1 -> Speed_OUT/1
  AccelResSw_IN/1 -> Assumption/1
  CoastSetSw_IN/1 -> CoastSetSw_OUT/1

== system CruiseControl_pp_harness_ReqProve/Test Unit (copied from CruiseControl_pp)/Input_Constraints/Assum_none ==
  CruiseOnOff_IN : Inport  OutDataTypeStr=boolean  PortDimensions=1
  Brake_IN : Inport  Port=2  OutDataTypeStr=boolean  PortDimensions=1
  Speed_IN : Inport  Port=3  OutDataTypeStr=uint8  PortDimensions=1
  CoastSetSw_IN : Inport  Port=4  OutDataTypeStr=boolean  PortDimensions=1
  AccelResSw_IN : Inport  Port=5  OutDataTypeStr=boolean  PortDimensions=1
  CruiseOnOff_OUT : Outport
  Brake_OUT : Outport  Port=2
  Speed_OUT : Outport  Port=3
  CoastSetSw_OUT : Outport  Port=4
  AccelResSw_OUT : Outport  Port=5
  wires:
  CruiseOnOff_IN/1 -> CruiseOnOff_OUT/1
  Brake_IN/1 -> Brake_OUT/1
  Speed_IN/1 -> Speed_OUT/1
  AccelResSw_IN/1 -> AccelResSw_OUT/1
  CoastSetSw_IN/1 -> CoastSetSw_OUT/1

== system CruiseControl_pp_harness_ReqProve/Test Unit (copied from CruiseControl_pp)/Input_Constraints/Assum_tspeed_LE_90 ==
  CruiseOnOff_IN : Inport  OutDataTypeStr=boolean  PortDimensions=1
  Brake_IN : Inport  Port=2  OutDataTypeStr=boolean  PortDimensions=1
  Speed_IN : Inport  Port=3  OutDataTypeStr=uint8  PortDimensions=1
  CoastSetSw_IN : Inport  Port=4  OutDataTypeStr=boolean  PortDimensions=1
  AccelResSw_IN : Inport  Port=5  OutDataTypeStr=boolean  PortDimensions=1
  CruiseOnOff_OUT : Outport
  Brake_OUT : Outport  Port=2
  Speed_OUT : Outport  Port=3
  CoastSetSw_OUT : Outport  Port=4
  AccelResSw_OUT : Outport  Port=5
  wires:
  Speed_IN/1 -> Speed_OUT/1
  CoastSetSw_IN/1 -> CoastSetSw_OUT/1
  AccelResSw_IN/1 -> AccelResSw_OUT/1
  Brake_IN/1 -> Brake_OUT/1
  CruiseOnOff_IN/1 -> CruiseOnOff_OUT/1

== system CruiseControl_pp_harness_ReqProve/Test Unit (copied from CruiseControl_pp)/Field_Issue_Behavior/Prop_coast_pulse_eml/MATLAB Function ==
  engaged : Inport
  CoastSetSw : Inport  Port=2
  tspeed : Inport  Port=3
  " Demux " : Demux  Outputs=1
  " SFunction " : S-Function  Tag=Stateflow S-Function propertyLib 2  FunctionName=sf_sfun  PortCounts=[3 2]  SFunctionDeploymentMode=off  EnableBusSupport=off
  " Terminator " : Terminator
  property : Outport
  wires:
  " SFunction "/1 -> " Demux "/1
  " Demux "/1 -> " Terminator "/1
  " SFunction "/2 -> property/1  "property"
  tspeed/1 -> " SFunction "/3
  CoastSetSw/1 -> " SFunction "/2
  engaged/1 -> " SFunction "/1
